simulink model "NewDesignTECS"  (R2017b)
settings: Solver=FixedStepAuto  StartTime=0.0  StopTime=10.0  RelTol=1e-3
undefined symbols (not defined in the file): dt, g, hgt_error_gain, hgt_gain_ff, max_climb_rate, max_sink_rate, min_sink_rate, Pitch_Kd, Pitch_Ki, pitch_sp_limit, pitch_time_constant, SKE_weighting, SPE_weighting, speed_error_gain, STE_rate_max, STE_rate_min, STE_to_throttle, THR_Kd, THR_Ki, throttle_cruise, z0
settings Model: Creator=ken  LastModifiedBy=ken

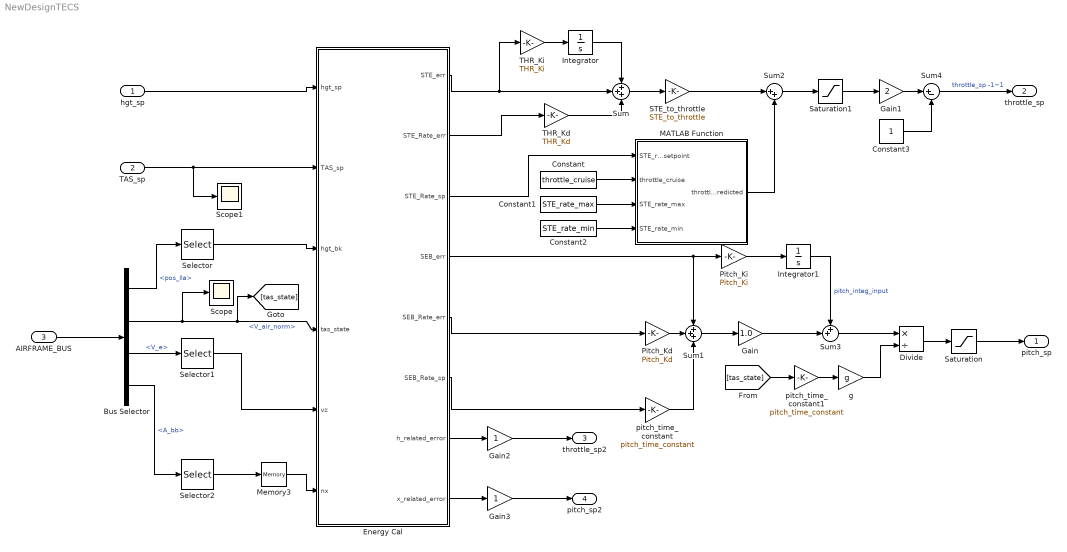
== system NewDesignTECS ==
  hgt_sp : Inport
  TAS_sp : Inport  Port=2
  AIRFRAME_BUS : Inport  Port=3  OutDataTypeStr=Bus: airframe
  Bus Selector : BusSelector  OutputSignals=pos_lla,V_air_norm,V_e,A_bb
  Constant : Constant  Value=throttle_cruise
  Constant1 : Constant  Value=STE_rate_max
  Constant2 : Constant  Value=STE_rate_min
  Constant3 : Constant
  Divide : Product  Inputs=*/
  Energy Cal : Subsystem
  Gain : Gain  Gain=1.0
  Gain1 : Gain  Gain=2
  Gain2 : Gain
  Gain3 : Gain
  Integrator : Integrator
  Integrator1 : Integrator
  MATLAB Function : MATLAB Function  TreatAsAtomicUnit=on
  Memory3 : Memory
  Pitch_Kd : Gain  Gain=Pitch_Kd
  Pitch_Ki : Gain  Gain=Pitch_Ki
  STE_to_throttle : Gain  Gain=STE_to_throttle
  Saturation : Saturate  UpperLimit=pitch_sp_limit  LowerLimit=-pitch_sp_limit
  Saturation1 : Saturate  UpperLimit=1  LowerLimit=0
  Scope : Scope
  Scope1 : Scope
  Selector : Selector  InputPortWidth=3  IndexOptions=Index vector (dialog)  Indices=3  OutputSizes=1
  Selector1 : Selector  InputPortWidth=3  IndexOptions=Index vector (dialog)  Indices=3  OutputSizes=1
  Selector2 : Selector  InputPortWidth=3  IndexOptions=Index vector (dialog)  Indices=1  OutputSizes=1
  Sum : Sum  Inputs=+++
  Sum1 : Sum  Inputs=+++
  Sum2 : Sum  Inputs=|++
  Sum3 : Sum  Inputs=++|
  Sum4 : Sum  Inputs=|+-
  THR_Kd : Gain  Gain=THR_Kd
  THR_Ki : Gain  Gain=THR_Ki
  g : Gain  Gain=g
  pitch_time_constant : Gain  Gain=pitch_time_constant
  pitch_time_constant1 : Gain  Gain=pitch_time_constant
  pitch_sp : Outport
  throttle_sp : Outport  Port=2  OutMin=0  OutMax=1  PortDimensions=1
  throttle_sp2 : Outport  Port=3
  pitch_sp2 : Outport  Port=4
  wires:
  Energy Cal/4(SEB_err) -> Pitch_Ki/1, Sum1/1
  Sum3/1 -> Divide/1
  Energy Cal/3(STE_Rate_sp) -> MATLAB Function/1(STE_rate_setpoint)
  Pitch_Kd/1 -> Sum1/2
  Integrator/1 -> Sum/1
  Pitch_Ki/1 -> Integrator1/1
  Gain1/1 -> Sum4/1
  STE_to_throttle/1 -> Sum2/1
  Constant2/1 -> MATLAB Function/4(STE_rate_min)
  Constant1/1 -> MATLAB Function/3(STE_rate_max)
  THR_Kd/1 -> Sum/3
  Selector1/1 -> Energy Cal/5(vz)
  Bus Selector/2 -> Scope/1, [tas_state], Energy Cal/4(tas_state)  "<V_air_norm>"
  Constant3/1 -> Sum4/2
  Energy Cal/2(STE_Rate_err) -> THR_Kd/1
  [tas_state] -> pitch_time_constant1/1
  Memory3/1 -> Energy Cal/6(nx)
  pitch_time_constant1/1 -> g/1
  g/1 -> Divide/2
  Energy Cal/6(SEB_Rate_sp) -> pitch_time_constant/1
  Divide/1 -> Saturation/1
  MATLAB Function/1(throttle_predicted) -> Sum2/2
  Bus Selector/3 -> Selector1/1  "<V_e>"
  Selector2/1 -> Memory3/1
  hgt_sp/1 -> Energy Cal/1(hgt_sp)
  Selector/1 -> Energy Cal/3(hgt_bk)
  AIRFRAME_BUS/1 -> Bus Selector/1
  Saturation/1 -> pitch_sp/1
  Gain/1 -> Sum3/2
  pitch_time_constant/1 -> Sum1/3
  Sum/1 -> STE_to_throttle/1
  Energy Cal/5(SEB_Rate_err) -> Pitch_Kd/1
  TAS_sp/1 -> Scope1/1, Energy Cal/2(TAS_sp)
  Sum1/1 -> Gain/1
  Sum4/1 -> throttle_sp/1  "throttle_sp -1~1"
  Bus Selector/1 -> Selector/1  "<pos_lla>"
  Bus Selector/4 -> Selector2/1  "<A_bb>"
  Integrator1/1 -> Sum3/1  "pitch_integ_input"
  Saturation1/1 -> Gain1/1
  Sum2/1 -> Saturation1/1
  Energy Cal/1(STE_err) -> Sum/2, THR_Ki/1
  THR_Ki/1 -> Integrator/1
  Constant/1 -> MATLAB Function/2(throttle_cruise)
  Energy Cal/7(h_related_error) -> Gain2/1
  Energy Cal/8(x_related_error) -> Gain3/1
  Gain2/1 -> throttle_sp2/1
  Gain3/1 -> pitch_sp2/1

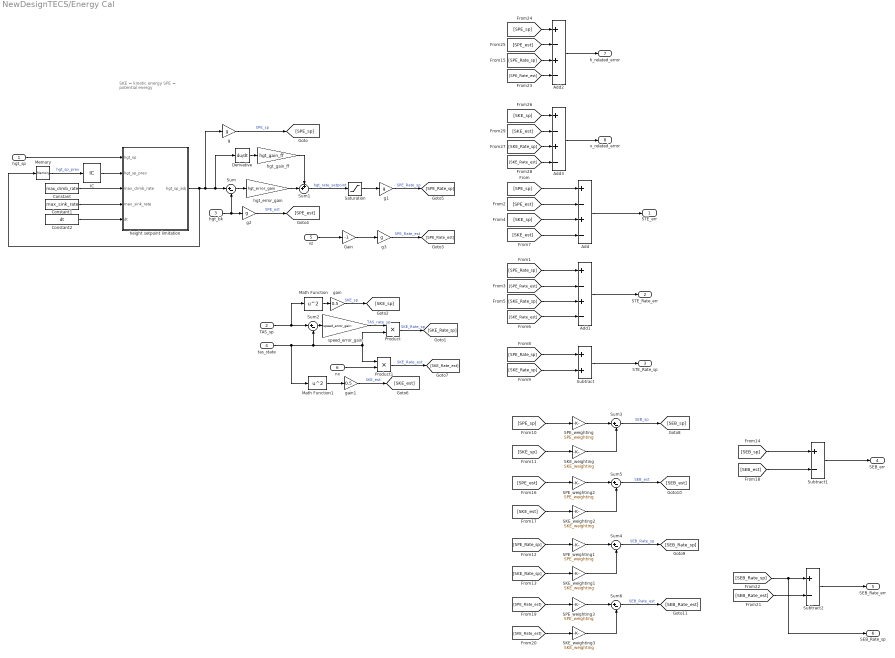
== system NewDesignTECS/Energy Cal ==
  note: SKE = kinetic energy
      | SPE = potential energy
  hgt_sp : Inport
  TAS_sp : Inport  Port=2
  hgt_bk : Inport  Port=3
  tas_state : Inport  Port=4
  vz : Inport  Port=5
  nx : Inport  Port=6
  Add{,1..3} (4 alike) : Sum  Inputs=+-+-
  Constant : Constant  Value=max_climb_rate
  Constant1 : Constant  Value=max_sink_rate
  Constant2 : Constant  Value=dt
  Derivative : Derivative
  Gain : Gain  Gain=-1
  IC : InitialCondition  Value=-z0
  Math Function : Math  Operator=square  SaturateOnIntegerOverflow=on
  Math Function1 : Math  Operator=square  SaturateOnIntegerOverflow=on
  Memory : Memory
  Product : Product
  Product1 : Product
  SKE_weighting{,1..3} (4 alike) : Gain  Gain=SKE_weighting
  SPE_weighting{,1..3} (4 alike) : Gain  Gain=SPE_weighting
  Saturation : Saturate  UpperLimit=max_climb_rate  LowerLimit=-min_sink_rate
  Subtract : Sum
  Subtract1 : Sum  Inputs=+-
  Subtract2 : Sum  Inputs=+-
  Sum{,2..6} (6 alike) : Sum  Inputs=|+-
  Sum1 : Sum  Inputs=++|
  g{,1..3} (4 alike) : Gain  Gain=g
  gain : Gain  Gain=0.5
  gain1 : Gain  Gain=0.5
  height setpoint limitation : MATLAB Function  TreatAsAtomicUnit=on
  hgt_error_gain : Gain  Gain=hgt_error_gain
  hgt_gain_ff : Gain  Gain=hgt_gain_ff
  speed_error_gain : Gain  Gain=speed_error_gain
  STE_err : Outport
  STE_Rate_err : Outport  Port=2
  STE_Rate_sp : Outport  Port=3
  SEB_err : Outport  Port=4
  SEB_Rate_err : Outport  Port=5
  SEB_Rate_sp : Outport  Port=6
  h_related_error : Outport  Port=7
  x_related_error : Outport  Port=8
  wires:
  [SKE_est] -> Add/4
  vz/1 -> Gain/1
  Add1/1 -> STE_Rate_err/1
  hgt_error_gain/1 -> Sum1/2
  [SKE_Rate_est] -> Add1/4
  g1/1 -> [SPE_Rate_sp]  "SPE_Rate_sp"
  Derivative/1 -> hgt_gain_ff/1
  g/1 -> [SPE_sp]  "SPE_sp"
  Product1/1 -> [SKE_Rate_est]  "SKE_Rate_est"
  speed_error_gain/1 -> Product/1  "TAS_rate_sp"
  g2/1 -> [SPE_est]  "SPE_est"
  g3/1 -> [SPE_Rate_est]  "SPE_Rate_est"
  Sum/1 -> hgt_error_gain/1
  gain/1 -> [SKE_sp]  "SKE_sp"
  Math Function1/1 -> gain1/1
  [SPE_Rate_sp] -> Add1/1
  hgt_gain_ff/1 -> Sum1/1
  Math Function/1 -> gain/1
  gain1/1 -> [SKE_est]  "SKE_est"
  Product/1 -> [SKE_Rate_sp]  "SKE_Rate_sp"
  nx/1 -> Product1/2
  [SKE_Rate_sp] -> Add1/3
  [SKE_sp] -> Add/3
  Gain/1 -> g3/1
  Sum2/1 -> speed_error_gain/1
  Sum1/1 -> Saturation/1  "hgt_rate_setpoint"
  [SPE_est] -> Add/2
  [SPE_Rate_est] -> Add1/2
  hgt_bk/1 -> Sum/2, g2/1
  tas_state/1 -> Sum2/2, Product/2, Product1/1, Math Function1/1
  TAS_sp/1 -> Math Function/1, Sum2/1
  Add/1 -> STE_err/1
  [SPE_sp] -> Add/1
  [SPE_Rate_sp] -> Subtract/1
  [SKE_Rate_sp] -> Subtract/2
  Subtract/1 -> STE_Rate_sp/1
  [SPE_sp] -> SPE_weighting/1
  SPE_weighting/1 -> Sum3/1
  [SKE_sp] -> SKE_weighting/1
  SKE_weighting/1 -> Sum3/2
  Sum3/1 -> [SEB_sp]  "SEB_sp"
  [SKE_Rate_sp] -> SKE_weighting1/1
  SKE_weighting1/1 -> Sum4/2
  [SPE_Rate_sp] -> SPE_weighting1/1
  Sum4/1 -> [SEB_Rate_sp]  "SEB_Rate_sp"
  SPE_weighting1/1 -> Sum4/1
  [SKE_est] -> SKE_weighting2/1
  SKE_weighting2/1 -> Sum5/2
  [SPE_est] -> SPE_weighting2/1
  SPE_weighting2/1 -> Sum5/1
  Sum5/1 -> [SEB_est]  "SEB_est"
  SKE_weighting3/1 -> Sum6/2
  [SPE_Rate_est] -> SPE_weighting3/1
  SPE_weighting3/1 -> Sum6/1
  [SKE_Rate_est] -> SKE_weighting3/1
  Sum6/1 -> [SEB_Rate_est]  "SEB_Rate_est"
  [SEB_sp] -> Subtract1/1
  [SEB_est] -> Subtract1/2
  Subtract1/1 -> SEB_err/1
  [SEB_Rate_sp] -> SEB_Rate_sp/1, Subtract2/1
  [SEB_Rate_est] -> Subtract2/2
  Subtract2/1 -> SEB_Rate_err/1
  height setpoint limitation/1(hgt_sp_adj) -> Sum/1, Derivative/1, g/1, Memory/1
  Saturation/1 -> g1/1
  Constant/1 -> height setpoint limitation/3(max_climb_rate)
  Constant2/1 -> height setpoint limitation/5(dt)
  Constant1/1 -> height setpoint limitation/4(max_sink_rate)
  Memory/1 -> IC/1  "hgt_sp_prev"
  IC/1 -> height setpoint limitation/2(hgt_sp_prev)
  hgt_sp/1 -> height setpoint limitation/1(hgt_sp)
  [SPE_sp] -> Add2/1
  [SPE_est] -> Add2/2
  [SPE_Rate_sp] -> Add2/3
  [SPE_Rate_est] -> Add2/4
  Add2/1 -> h_related_error/1
  [SKE_sp] -> Add3/1
  [SKE_est] -> Add3/2
  [SKE_Rate_sp] -> Add3/3
  [SKE_Rate_est] -> Add3/4
  Add3/1 -> x_related_error/1

== matlab function NewDesignTECS/Energy Cal/height setpoint limitation ==
  data: hgt_sp input; hgt_sp_adj output; hgt_sp_prev input; max_climb_rate input; max_sink_rate input; dt input
% limit the maximum height setpoint from current height depends on maximum
% climb rate, sind rate and dt.
function hgt_sp_adj = fcn(hgt_sp,hgt_sp_prev,max_climb_rate,max_sink_rate,dt)
if ((hgt_sp - hgt_sp_prev) > (max_climb_rate * dt)) 
	hgt_sp_adj = hgt_sp_prev + max_climb_rate * dt;
elseif ((hgt_sp - hgt_sp_prev) < (-max_sink_rate * dt))
	hgt_sp_adj = hgt_sp_prev - max_sink_rate * dt;
else
    hgt_sp_adj = hgt_sp;
	
end

== matlab function NewDesignTECS/MATLAB Function ==
  data: STE_rate_setpoint input; throttle_predicted output; throttle_cruise input; STE_rate_max input; STE_rate_min input
function throttle_predicted = fcn(STE_rate_setpoint,throttle_cruise,STE_rate_max,STE_rate_min)
if (STE_rate_setpoint >= 0) 
	throttle_predicted = throttle_cruise + STE_rate_setpoint / STE_rate_max * (1.0 - throttle_cruise);

else
    throttle_predicted = throttle_cruise + STE_rate_setpoint / STE_rate_min * (0.0 - throttle_cruise);
end
